simulink model "FCS_MPC_6ph_CIL_FCS_reduced"  (R2022a)
settings: Solver=ode23t  StartTime=0.0  StopTime=0.1  RelTol=1e-3  AbsTol=1e-3  EnableMultiTasking=on
values from neighbouring files (symbols this model uses):
  f_c = 100000    [Params_testbench.m]
  L_d = 0.0001473    [Params_testbench.m]
  L_q = 0.0001484    [Params_testbench.m]
  L_x = 0.00005566    (= 5.566e-05)    [Params_testbench.m]
  L_y = L_x    (= 5.566e-05)    [Params_testbench.m]
  p = 5    [Params_testbench.m]
  psi_pm = 0.0048    [Params_testbench.m]
  R_ph = 0.1278    [Params_testbench.m]
  u_dc = 36.0    (= 36)    [Params_testbench.m]
libraries: nesl_utility x39, fl_lib x32, hdlsllib x20, ee_lib x12, simulink x2, spsAlphaBetaZerotodq0Lib x1
(part 2 of 3)

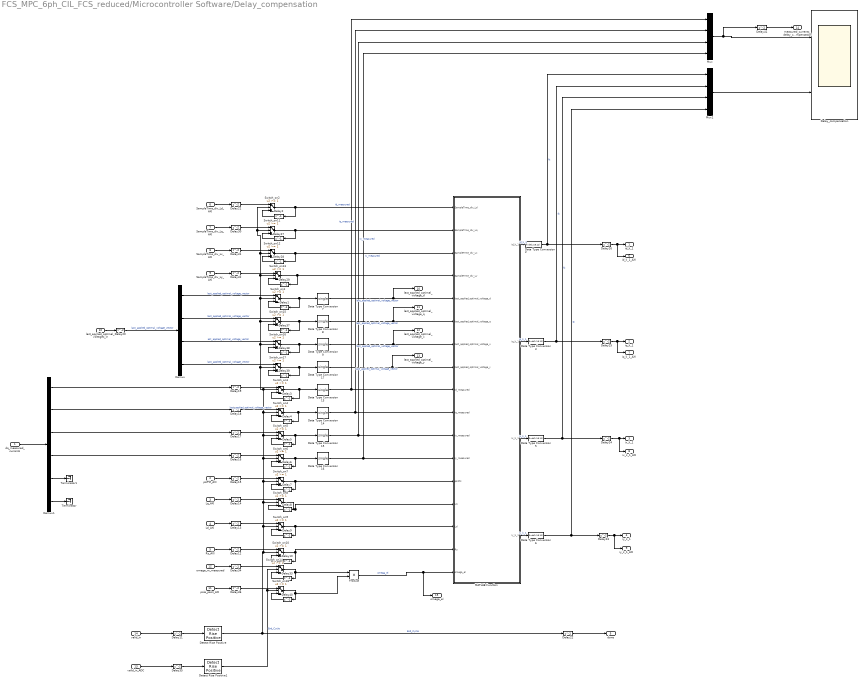
== system FCS_MPC_6ph_CIL_FCS_reduced/Microcontroller Software/Delay_compensation ==
  dq_measured_currents : Inport
  psiPM_AXI : Inport  Port=2
  Lq_AXI : Inport  Port=3
  Ld_AXI : Inport  Port=4
  Rs_AXI : Inport  Port=5
  SampleTime_div_Ld_AXI : Inport  Port=6
  SampleTime_div_Lq_AXI : Inport  Port=7
  SampleTime_div_Lx_AXI : Inport  Port=8
  SampleTime_div_Ly_AXI : Inport  Port=9
  last_applied_optimal_voltages_in : Inport  Port=10
  pole_pairs_AXI : Inport  Port=11
  omega_m_measured : Inport  Port=12
  valid_in_ADC : Inport  Port=13
  valid_in : Inport  Port=14
  Data Type Conversion{7..9,13..17} (8 alike) : DataTypeConversion  OutDataTypeStr=single  RndMeth=Nearest  SaturateOnIntegerOverflow=off
  Data Type Conversion{2..3,5..6} (4 alike) : DataTypeConversion  OutDataTypeStr=fixdt(1,18,11)  SaturateOnIntegerOverflow=off  RndMeth=Floor
  Delay{1..10,27..29,33,37..40} (18 alike) : Delay  DelayLength=1
  Delay{11..26,30..32,34..36,41} (23 alike) : Delay
  Delay_compensation : Scope  NumInputPorts=2
  Demux : Demux
  Demux1 : Demux  Outputs=6
  Detect Rise Positive : hdlsllib/Logic and Bit Operations/Detect Rise Positive  vinit=0  OutDataTypeStr=boolean
      settings: SourceProductBaseCode=SL
  Detect Rise Positive1 : hdlsllib/Logic and Bit Operations/Detect Rise Positive  vinit=0  OutDataTypeStr=boolean
      settings: SourceProductBaseCode=SL
  MATLAB Function : MATLAB Function  TreatAsAtomicUnit=on  SystemSampleTime=1/100000000
  Mux : Mux
  Mux1 : Mux
  Product : Product  Inputs=**
  Switch_on{1..18} (18 alike) : Switch  Threshold=1  RndMeth=Simplest  SaturateOnIntegerOverflow=off  InputSameDT=off  OutDataTypeStr=Inherit: Same as first input
  Terminator : Terminator
  Terminator1 : Terminator
  id_k_1 : Outport
  iq_k_1 : Outport  Port=2
  ix_k_1 : Outport  Port=3
  iy_k_1 : Outport  Port=4
  done : Outport  Port=5
  id_k_1_AXI : Outport  Port=6
  iq_k_1_AXI : Outport  Port=7
  ix_k_1_AXI : Outport  Port=8
  iy_k_1_AXI : Outport  Port=9
  last_applied_optimal_voltage_d : Outport  Port=10
  last_applied_optimal_voltage_q : Outport  Port=11
  last_applied_optimal_voltage_x : Outport  Port=12
  last_applied_optimal_voltage_y : Outport  Port=13
  measured_currents_delay_compensation : Outport  Port=14
  omega_el : Outport  Port=15
  wires:
  Delay33/1 -> Switch_on14/3
  pole_pairs_AXI/1 -> Delay36/1
  Delay9/1 -> Switch_on9/3
  Switch_on9/1 -> Delay9/1, MATLAB Function/15(Ld)
  Delay32/1 -> Switch_on13/1
  Lq_AXI/1 -> Delay14/1
  Delay31/1 -> Switch_on12/1
  Switch_on12/1 -> Delay28/1, MATLAB Function/3(SampleTime_div_Lx)
  Delay30/1 -> Switch_on11/1
  Delay29/1 -> Switch_on13/3
  SampleTime_div_Lx_AXI/1 -> Delay31/1
  Delay26/1 -> id_k_1_AXI/1, id_k_1/1
  Product/1 -> omega_el/1, MATLAB Function/17(omega_el)  "omega_el"
  Delay11/1 -> Detect Rise Positive/1
  Delay2/1 -> Switch_on2/3
  SampleTime_div_Lq_AXI/1 -> Delay30/1
  Switch_on5/1 -> Delay5/1, Data Type Conversion15/1
  Delay12/1 -> Switch_on10/1
  Rs_AXI/1 -> Delay12/1
  Delay1/1 -> Switch_on1/3
  Delay27/1 -> Switch_on11/3
  Delay21/1 -> Switch_on2/1
  Delay23/1 -> iy_k_1_AXI/1, iy_k_1/1
  Delay24/1 -> ix_k_1_AXI/1, ix_k_1/1
  Delay20/1 -> Demux/1  "last_applied_optimal_voltage_vector"
  Switch_on1/1 -> Delay1/1, Data Type Conversion7/1
  Delay8/1 -> Switch_on8/3
  Delay10/1 -> Switch_on10/3
  valid_in/1 -> Delay11/1
  Switch_on6/1 -> Delay6/1, Data Type Conversion16/1
  psiPM_AXI/1 -> Delay15/1
  Delay25/1 -> iq_k_1_AXI/1, iq_k_1/1
  Switch_on13/1 -> Delay29/1, MATLAB Function/4(SampleTime_div_Ly)
  Switch_on4/1 -> Delay4/1, Data Type Conversion14/1
  Delay15/1 -> Switch_on7/1
  SampleTime_div_Ly_AXI/1 -> Delay32/1
  Switch_on10/1 -> Delay10/1, MATLAB Function/16(Rs)
  Delay7/1 -> Switch_on7/3
  Delay28/1 -> Switch_on12/3
  Switch_on8/1 -> Delay8/1, MATLAB Function/14(Lq)
  Ld_AXI/1 -> Delay13/1
  Delay6/1 -> Switch_on6/3
  Delay4/1 -> Switch_on4/3
  Switch_on11/1 -> Delay27/1, MATLAB Function/2(SampleTime_div_Lq)
  Delay3/1 -> Switch_on3/3
  Delay14/1 -> Switch_on8/1
  Switch_on2/1 -> Delay2/1, MATLAB Function/1(SampleTime_div_Ld)
  Delay22/1 -> done/1
  Switch_on3/1 -> Delay3/1, Data Type Conversion13/1
  Delay13/1 -> Switch_on9/1
  Delay5/1 -> Switch_on5/3
  SampleTime_div_Ld_AXI/1 -> Delay21/1
  last_applied_optimal_voltages_in/1 -> Delay20/1
  omega_m_measured/1 -> Delay34/1
  Delay35/1 -> Detect Rise Positive1/1
  valid_in_ADC/1 -> Delay35/1
  Delay34/1 -> Switch_on14/1
  Delay36/1 -> Switch_on18/1
  Delay37/1 -> Switch_on15/3
  Delay38/1 -> Switch_on16/3
  Switch_on16/1 -> Data Type Conversion9/1, Delay38/1
  Delay39/1 -> Switch_on17/3
  Detect Rise Positive/1 -> Switch_on17/2, Switch_on16/2, Switch_on15/2, Switch_on13/2, Switch_on2/2, Switch_on11/2, Switch_on12/2, Switch_on1/2, Switch_on3/2, Switch_on4/2, Switch_on5/2, Switch_on6/2, Switch_on7/2, Switch_on8/2, Switch_on9/2, Switch_on10/2, Delay22/1  "End_Cycle"
  Switch_on17/1 -> Data Type Conversion17/1, Delay39/1
  Delay19/1 -> Switch_on3/1
  Delay18/1 -> Switch_on4/1  "last_applied_optimal_voltage_vector"
  Delay17/1 -> Switch_on5/1
  Delay16/1 -> Switch_on6/1
  Switch_on14/1 -> Product/1, Delay33/1
  MATLAB Function/1(id_k_1) -> Data Type Conversion2/1  "id_k_1"
  MATLAB Function/2(iq_k_1) -> Data Type Conversion3/1  "iq_k_1"
  MATLAB Function/3(ix_k_1) -> Data Type Conversion5/1  "ix_k_1"
  MATLAB Function/4(iy_k_1) -> Data Type Conversion6/1  "iy_k_1"
  Switch_on18/1 -> Product/2, Delay40/1
  Detect Rise Positive1/1 -> Switch_on18/2, Switch_on14/2  "End_Cycle"
  Delay40/1 -> Switch_on18/3
  Data Type Conversion13/1 -> Mux/1, MATLAB Function/9(id_measured)  "id_measured"
  Data Type Conversion14/1 -> Mux/2, MATLAB Function/10(iq_measured)  "iq_measured"
  Data Type Conversion15/1 -> Mux/3, MATLAB Function/11(ix_measured)  "ix_measured"
  Data Type Conversion16/1 -> Mux/4, MATLAB Function/12(iy_measured)  "iy_measured"
  Switch_on7/1 -> MATLAB Function/13(psiPM), Delay7/1
  Mux/1 -> Delay41/1, Delay_compensation/1
  Mux1/1 -> Delay_compensation/2
  Switch_on15/1 -> Data Type Conversion8/1, Delay37/1
  Demux/1 -> Switch_on1/1  "last_applied_optimal_voltage_vector"
  Demux/2 -> Switch_on15/1  "last_applied_optimal_voltage_vector"
  Demux/3 -> Switch_on16/1  "ast_applied_optimal_voltage_vector"
  Demux/4 -> Switch_on17/1  "last_applied_optimal_voltage_vector"
  Data Type Conversion2/1 -> Mux1/1, Delay26/1  "fc"
  Data Type Conversion3/1 -> Mux1/2, Delay25/1  "fc"
  Data Type Conversion5/1 -> Mux1/3, Delay24/1  "fc"
  Data Type Conversion6/1 -> Mux1/4, Delay23/1  "fc"
  Data Type Conversion7/1 -> last_applied_optimal_voltage_d/1, MATLAB Function/5(last_applied_optimal_voltage_d)  "last_applied_optimal_voltage_vector"
  Data Type Conversion8/1 -> last_applied_optimal_voltage_q/1, MATLAB Function/6(last_applied_optimal_voltage_q)  "last_applied_optimal_voltage_vector"
  Data Type Conversion9/1 -> last_applied_optimal_voltage_x/1, MATLAB Function/7(last_applied_optimal_voltage_x)  "last_applied_optimal_voltage_vector"
  Data Type Conversion17/1 -> last_applied_optimal_voltage_y/1, MATLAB Function/8(last_applied_optimal_voltage_y)  "last_applied_optimal_voltage_vector"
  Delay41/1 -> measured_currents_delay_compensation/1
  dq_measured_currents/1 -> Demux1/1
  Demux1/6 -> Terminator/1
  Demux1/5 -> Terminator1/1
  Demux1/1 -> Delay19/1
  Demux1/2 -> Delay18/1
  Demux1/3 -> Delay17/1
  Demux1/4 -> Delay16/1

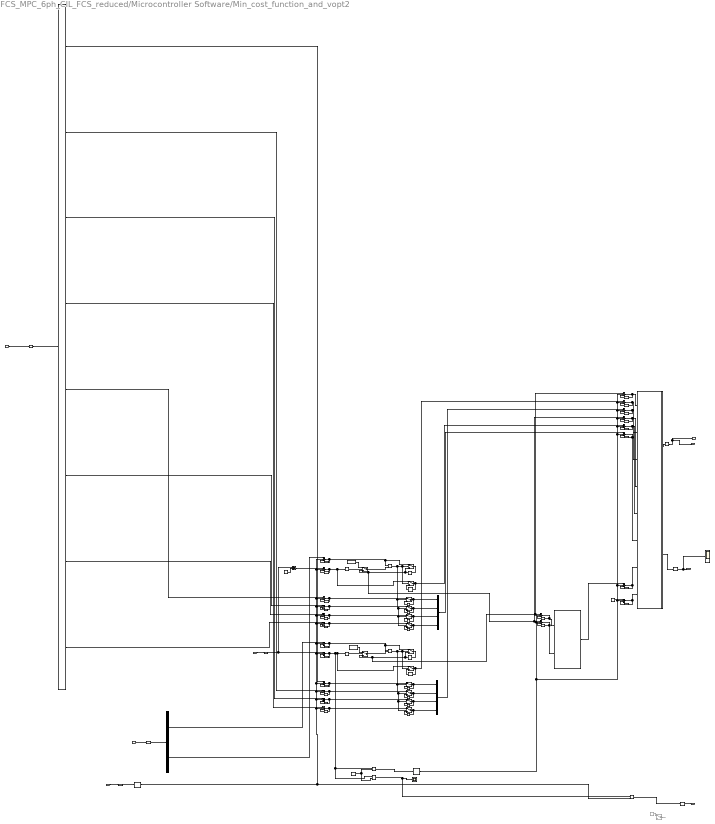
== system FCS_MPC_6ph_CIL_FCS_reduced/Microcontroller Software/Min_cost_function_and_vopt2 ==
  note: fixdt(1,24,11)
  Index_in : Inport
  valid_in : Inport  Port=2
  J_in : Inport  Port=3
  phase_voltages_per_switching_state_in : Inport  Port=4
  Add : Sum
  Compare To Constant : hdlsllib/Logic and Bit Operations/Compare To Constant  relop=<=  const=1  OutDataTypeStr=boolean
      settings: SourceProductBaseCode=SL
  Compare To Constant1 : hdlsllib/Logic and Bit Operations/Compare To Constant  relop=<=  const=9  OutDataTypeStr=boolean
      settings: SourceProductBaseCode=SL
  Constant : Constant  Value=1000  OutDataTypeStr=fixdt(1,20,9)  SampleTime=-1
  Constant1 : Constant  Value=8  OutDataTypeStr=int32  SampleTime=-1
  Constant11 : Constant  Value=[0;0;0;0]  OutDataTypeStr=fixdt(1,24,11)  SampleTime=-1
  Constant18 : Constant  Value=8  OutDataTypeStr=int32  SampleTime=-1
  Constant2 : Constant  Commented=on  Value=0  OutDataTypeStr=boolean  SampleTime=-1
  Constant3 : Constant  Value=1000  OutDataTypeStr=fixdt(1,20,9)  SampleTime=-1
  Delay{,1..5,9,15,17..23,25..26,34..43,56..57,68..71,371..372} (35 alike) : Delay  DelayLength=1
  Delay10 : Delay  DelayLength=3
  Delay11 : Delay  DelayLength=3
  Delay12 : Delay  DelayLength=3
  Delay6 : Delay
  Delay7 : Delay
  Delay8 : Delay
  Delay_compensation_test1 : Scope
  Demux : Demux  Outputs=2
  Demux1 : Demux  Outputs=8
  Detect Rise Positive : hdlsllib/Logic and Bit Operations/Detect Rise Positive  vinit=0  OutDataTypeStr=boolean
      settings: SourceProductBaseCode=SL
  Detect Rise Positive1 : hdlsllib/Logic and Bit Operations/Detect Rise Positive  vinit=0  OutDataTypeStr=boolean
      settings: SourceProductBaseCode=SL
  Logical Operator : Logic  AllPortsSameDT=off  OutDataTypeStr=boolean
  MATLAB Function : MATLAB Function  TreatAsAtomicUnit=on  SystemSampleTime=1/100000000
  MinMax : MinMax  Inputs=2  ZeroCross=off
  Mux : Mux
  Mux1 : Mux
  Relational Operator : RelationalOperator  Operator=<  OutDataTypeStr=boolean  RndMeth=Simplest  InputSameDT=off
  Relational Operator1 : RelationalOperator  Operator=<  OutDataTypeStr=boolean  RndMeth=Simplest  InputSameDT=off
  Relational Operator2 : RelationalOperator  Operator=<  OutDataTypeStr=boolean  RndMeth=Simplest  InputSameDT=off
  Relational Operator9 : RelationalOperator  OutDataTypeStr=boolean  RndMeth=Simplest  InputSameDT=off
  Scope : Scope
  Switch{,1,3..6,8..9,11..14} (12 alike) : Switch  Criteria=u2 > Threshold  SaturateOnIntegerOverflow=off  InputSameDT=off  OutDataTypeStr=Inherit: Same as first input
  Switch10 : Switch  Criteria=u2 > Threshold  OutDataTypeStr=int32  SaturateOnIntegerOverflow=off  InputSameDT=off
  Switch2 : Switch  Criteria=u2 > Threshold  OutDataTypeStr=int32  SaturateOnIntegerOverflow=off  InputSameDT=off
  Switch7 : Switch  Commented=on  Criteria=u2 > Threshold  SaturateOnIntegerOverflow=off  InputSameDT=off
  Switch_on{1..13,51,70..75,98..99} (22 alike) : Switch  Threshold=1  RndMeth=Simplest  SaturateOnIntegerOverflow=off  InputSameDT=off  OutDataTypeStr=Inherit: Same as first input
  done : Outport
  Index : Outport  Port=2
  voltages : Outport  Port=3
  Index_AXI : Outport  Port=4
  wires:
  Demux/1 -> Switch_on4/1  "End_Cycle"
  Demux1/1 -> Switch_on2/1  "End_Cycle"
  Demux1/2 -> Switch_on3/1  "End_Cycle"
  Switch5/1 -> Mux/3, Delay4/1
  Delay3/1 -> Switch4/3
  Relational Operator/1 -> Switch5/2, Switch6/2, Switch4/2, Switch3/2, Switch2/2, Switch1/2
  Compare To Constant/1 -> Switch/2
  Switch1/1 -> Delay/1
  Switch6/1 -> Delay5/1, Mux/4
  Delay4/1 -> Switch5/3
  Switch4/1 -> Mux/2, Delay3/1
  Switch/1 -> Relational Operator/2
  Delay1/1 -> Switch2/3
  Delay5/1 -> Switch6/3
  Switch3/1 -> Mux/1, Delay2/1
  Delay2/1 -> Switch3/3
  Constant/1 -> Switch/1
  Switch_on4/1 -> Relational Operator/1, Switch1/1, Delay17/1
  Switch_on1/1 -> Delay18/1, Compare To Constant/1, Switch2/1, Relational Operator9/1, Relational Operator1/1
  Switch_on2/1 -> Delay19/1, Switch3/1
  Switch_on3/1 -> Delay20/1, Switch4/1
  Switch_on5/1 -> Switch5/1, Delay21/1
  Switch_on6/1 -> Switch6/1, Delay22/1
  valid_in/1 -> Delay6/1  "End_Cycle"
  Delay17/1 -> Switch_on4/3
  Delay18/1 -> Switch_on1/3
  Delay19/1 -> Switch_on2/3
  Delay20/1 -> Switch_on3/3
  Delay21/1 -> Switch_on5/3
  Delay22/1 -> Switch_on6/3
  Constant1/1 -> Relational Operator9/2, Relational Operator1/2
  Constant2/1 -> Switch7/1
  Demux1/3 -> Switch_on5/1  "End_Cycle"
  Demux1/4 -> Switch_on6/1  "End_Cycle"
  Demux/2 -> Switch_on10/1  "End_Cycle"
  Delay34/1 -> Switch_on10/3
  Switch8/1 -> Relational Operator2/2
  Switch_on8/1 -> Delay36/1, Switch11/1
  Demux1/6 -> Switch_on9/1  "End_Cycle"
  Delay26/1 -> Switch10/3
  Add/1 -> Switch_on7/1
  Delay36/1 -> Switch_on8/3
  Delay39/1 -> Switch_on11/3
  Switch_on7/1 -> Delay35/1, Switch10/1, Compare To Constant1/1
  Compare To Constant1/1 -> Switch8/2
  Switch_on9/1 -> Delay38/1, Switch12/1
  Delay40/1 -> Switch_on12/3
  Delay35/1 -> Switch_on7/3
  Switch_on11/1 -> Switch13/1, Delay39/1
  Delay43/1 -> Switch14/3
  Switch_on12/1 -> Switch14/1, Delay40/1
  Delay37/1 -> Switch11/3
  Relational Operator2/1 -> Switch13/2, Switch14/2, Switch12/2, Switch11/2, Switch10/2, Switch9/2
  Switch9/1 -> Delay25/1
  Delay42/1 -> Switch13/3
  Demux1/5 -> Switch_on8/1  "End_Cycle"
  Demux1/7 -> Switch_on11/1  "End_Cycle"
  Switch_on10/1 -> Relational Operator2/1, Switch9/1, Delay34/1
  Demux1/8 -> Switch_on12/1  "End_Cycle"
  Delay38/1 -> Switch_on9/3
  Constant3/1 -> Switch8/1
  Delay41/1 -> Switch12/3
  Detect Rise Positive/1 -> Logical Operator/2, Switch_on10/2, Switch_on7/2, Switch_on8/2, Switch_on9/2, Switch_on11/2, Switch_on12/2, Switch_on4/2, Switch_on1/2, Switch_on2/2, Switch_on3/2, Switch_on5/2, Switch_on6/2  "End_Cycle"
  Constant18/1 -> Add/2
  Delay371/1 -> Switch_on98/3
  Switch_on98/1 -> Delay371/1, MinMax/1
  Switch_on99/1 -> Delay372/1, MinMax/2
  Delay372/1 -> Switch_on99/3
  Relational Operator1/1 -> Logical Operator/1, Scope/1  "End_Cycle"
  Switch13/1 -> Mux1/3, Delay42/1
  Switch12/1 -> Mux1/2, Delay41/1
  Switch14/1 -> Mux1/4, Delay43/1
  Switch11/1 -> Mux1/1, Delay37/1
  J_in/1 -> Delay7/1  "End_Cycle"
  phase_voltages_per_switching_state_in/1 -> Delay8/1  "End_Cycle"
  Logical Operator/1 -> Delay12/1
  Delay6/1 -> Detect Rise Positive/1
  Delay7/1 -> Demux/1
  Delay8/1 -> Demux1/1
  Index_in/1 -> Delay9/1
  Switch7/1 -> ?
  MATLAB Function/2(voltages) -> Delay11/1
  MATLAB Function/1(Index) -> Delay10/1
  Constant11/1 -> Switch_on13/1
  Switch_on13/1 -> MATLAB Function/8(voltages_default), Delay15/1
  Delay15/1 -> Switch_on13/3
  Switch_on51/1 -> MATLAB Function/7(min), Delay23/1
  Delay23/1 -> Switch_on51/3
  Switch_on70/1 -> MATLAB Function/6(voltages_2), Delay56/1
  Delay56/1 -> Switch_on70/3
  Switch10/1 -> Switch_on71/1, Delay26/1
  Switch_on71/1 -> MATLAB Function/5(Index_2), Delay57/1
  Delay57/1 -> Switch_on71/3
  Switch_on72/1 -> MATLAB Function/4(J_2), Delay68/1
  Delay68/1 -> Switch_on72/3
  Switch_on73/1 -> MATLAB Function/3(voltages_1), Delay69/1
  Delay69/1 -> Switch_on73/3
  Switch2/1 -> Switch_on74/1, Delay1/1
  Switch_on74/1 -> MATLAB Function/2(Index_1), Delay70/1
  Delay70/1 -> Switch_on74/3
  Switch_on75/1 -> MATLAB Function/1(J_1), Delay71/1
  Delay71/1 -> Switch_on75/3
  Delay/1 -> Switch_on75/1, Switch_on98/1, Switch/3, Switch1/3  "last_applied_optimal_voltage_vector"
  Mux/1 -> Switch_on73/1  "last_applied_optimal_voltage_vector"
  Delay25/1 -> Switch_on72/1, Switch_on99/1, Switch8/3, Switch9/3  "last_applied_optimal_voltage_vector"
  Mux1/1 -> Switch_on70/1  "last_applied_optimal_voltage_vector"
  MinMax/1 -> Switch_on51/1  "last_applied_optimal_voltage_vector"
  Delay10/1 -> Index_AXI/1, Index/1
  Delay11/1 -> Delay_compensation_test1/1, voltages/1
  Delay12/1 -> done/1
  Detect Rise Positive1/1 -> Switch_on75/2, Switch_on74/2, Switch_on73/2, Switch_on72/2, Switch_on71/2, Switch_on70/2, Switch_on51/2, Switch_on13/2, Switch_on98/2, Switch_on99/2  "End_Cycle"
  Relational Operator9/1 -> Detect Rise Positive1/1  "End_Cycle"
  Delay9/1 -> Switch_on1/1, Add/1

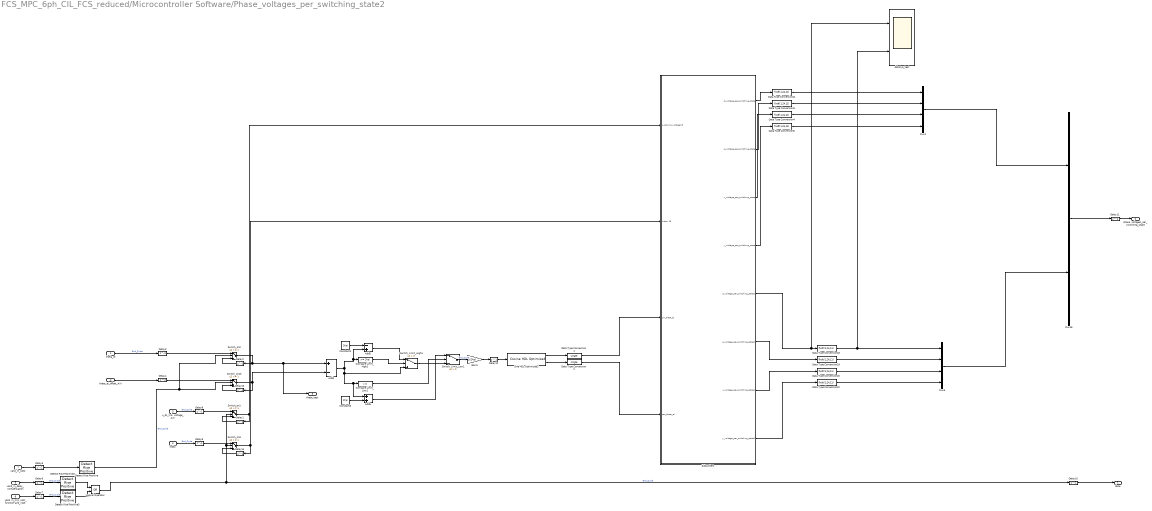
== system FCS_MPC_6ph_CIL_FCS_reduced/Microcontroller Software/Phase_voltages_per_switching_state2 ==
  theta_el : Inport
  theta_el_offset_AXI : Inport  Port=2
  u_dc_link_voltage_AXI : Inport  Port=3
  Index : Inport  Port=4
  valid_in_delay_compensation : Inport  Port=5
  valid_in_min_cost_function-and_vopt : Inport  Port=6
  valid_in_ADC : Inport  Port=7
  Add4 : Sum  Inputs=+-  OutDataTypeStr=Inherit: Same as first input
  Add5 : Sum  Inputs=-+  OutDataTypeStr=Inherit: Same as first input
  Add6 : Sum  OutDataTypeStr=Inherit: Same as first input
  Compare Limit_High1 : simulink/Logic and Bit Operations/Compare To Constant  relop=>=  const=2*pi  OutDataTypeStr=boolean
  Compare Limit_Low1 : simulink/Logic and Bit Operations/Compare To Constant  relop=<  const=0  OutDataTypeStr=boolean
  Constant2 : Constant  Value=2*pi  OutDataTypeStr=fixdt(1,18,14)  SampleTime=1/100000000
  Constant3 : Constant  Value=2*pi  OutDataTypeStr=fixdt(1,18,14)  SampleTime=1/100000000
  Data Type Conversion1 : DataTypeConversion  OutDataTypeStr=single  SaturateOnIntegerOverflow=off  RndMeth=Floor
  Data Type Conversion{3..5,18..22} (8 alike) : DataTypeConversion  OutDataTypeStr=fixdt(1,24,11)  SaturateOnIntegerOverflow=off  RndMeth=Floor
  Data Type Conversion2 : DataTypeConversion  OutDataTypeStr=single  SaturateOnIntegerOverflow=off  RndMeth=Floor
  Delay{1..2,6..14} (11 alike) : Delay  DelayLength=1
  Delay3 : Delay
  Delay4 : Delay
  Delay5 : Delay
  Detect Rise Positive : hdlsllib/Logic and Bit Operations/Detect Rise Positive  vinit=0  OutDataTypeStr=boolean
      settings: SourceProductBaseCode=SL
  Detect Rise Positive2 : hdlsllib/Logic and Bit Operations/Detect Rise Positive  vinit=0  OutDataTypeStr=boolean
      settings: SourceProductBaseCode=SL
  Detect Rise Positive3 : hdlsllib/Logic and Bit Operations/Detect Rise Positive  vinit=0  OutDataTypeStr=boolean
      settings: SourceProductBaseCode=SL
  Gain1 : Gain  Gain=1/(2*pi)  OutDataTypeStr=Inherit: Same as input  ParamDataTypeStr=Inherit: Same as input
  Logical Operator : Logic  Operator=OR  AllPortsSameDT=off  OutDataTypeStr=boolean
  Mux1 : Mux
  Mux16 : Mux  Inputs=2
  Mux5 : Mux
  Sine HDL Optimized2 : hdlsllib/Lookup Tables/Cosine HDL Optimized  OutputFormula=sin(2*pi*u) and cos(2*pi*u)  NumDataPoints=512  TableDataTypeStr=fixdt(1,15,14)  SimulateLUTROMDelay=off
      settings: SourceProductBaseCode=SL
  Subsystem : Subsystem
  Switch_Limit_High1 : Switch  Criteria=u2 > Threshold  SaturateOnIntegerOverflow=off  InputSameDT=off  OutDataTypeStr=Inherit: Same as first input
  Switch_Limit_Low1 : Switch  Criteria=u2 > Threshold  SaturateOnIntegerOverflow=off  InputSameDT=off  OutDataTypeStr=Inherit: Same as first input
  Switch_on1 : Switch  Threshold=1  OutDataTypeStr=single  RndMeth=Simplest  SaturateOnIntegerOverflow=off  InputSameDT=off
  Switch_on13 : Switch  Threshold=1  RndMeth=Simplest  SaturateOnIntegerOverflow=off  InputSameDT=off  OutDataTypeStr=Inherit: Same as first input
  Switch_on2 : Switch  Threshold=1  RndMeth=Simplest  SaturateOnIntegerOverflow=off  InputSameDT=off  OutDataTypeStr=Inherit: Same as first input
  Switch_on3 : Switch  Threshold=1  OutDataTypeStr=int32  RndMeth=Simplest  SaturateOnIntegerOverflow=off  InputSameDT=off
  datatyp_test : Scope  NumInputPorts=2
  done : Outport
  phase_voltages_per_switching_state : Outport  Port=2
  theta_test : Outport  Port=3
  wires:
  Delay14/1 -> Switch_on3/3
  Delay13/1 -> Switch_on13/3
  Switch_on13/1 -> Delay13/1, Add4/2
  u_dc_link_voltage_AXI/1 -> Delay8/1  "End_Cycle"
  Switch_on1/1 -> Subsystem/1(u_dc_link_voltage15), Delay1/1
  Logical Operator/1 -> Delay10/1, Switch_on3/2, Switch_on1/2  "End_Cycle"
  Delay1/1 -> Switch_on1/3
  Index/1 -> Delay9/1  "End_Cycle"
  Switch_on3/1 -> Delay14/1, Subsystem/2(Index 15)
  Mux1/1 -> Mux16/1
  Mux5/1 -> Mux16/2
  Mux16/1 -> Delay11/1
  valid_in_ADC/1 -> Delay5/1
  valid_in_delay_compensation/1 -> Delay6/1
  valid_in_min_cost_function-and_vopt/1 -> Delay7/1
  theta_el/1 -> Delay3/1  "End_Cycle"
  Add4/1 -> Switch_Limit_High1/3, Add6/1, Compare Limit_Low1/1, Add5/2, Compare Limit_High1/1
  Compare Limit_Low1/1 -> Switch_Limit_Low1/2
  Add5/1 -> Switch_Limit_High1/1
  theta_el_offset_AXI/1 -> Delay4/1
  Constant3/1 -> Add6/2
  Constant2/1 -> Add5/1
  Compare Limit_High1/1 -> Switch_Limit_High1/2
  Add6/1 -> Switch_Limit_Low1/1
  Switch_Limit_High1/1 -> Switch_Limit_Low1/3
  Delay2/1 -> Switch_on2/3
  Switch_on2/1 -> theta_test/1, Add4/1, Delay2/1
  Detect Rise Positive/1 -> Switch_on2/2, Switch_on13/2  "End_Cycle"
  Delay3/1 -> Switch_on2/1
  Delay4/1 -> Switch_on13/1
  Delay5/1 -> Detect Rise Positive/1
  Delay6/1 -> Detect Rise Positive2/1
  Delay7/1 -> Detect Rise Positive3/1
  Delay8/1 -> Switch_on1/1
  Delay9/1 -> Switch_on3/1
  Delay10/1 -> done/1
  Delay11/1 -> phase_voltages_per_switching_state/1
  Sine HDL Optimized2/2 -> Data Type Conversion2/1
  Subsystem/1(d_voltage_per_switching_state) -> Data Type Conversion21/1
  Subsystem/2(q_voltage_per_switching_state) -> Data Type Conversion3/1
  Subsystem/3(x_voltage_per_switching_state) -> Data Type Conversion4/1
  Subsystem/4(y_voltage_per_switching_state) -> Data Type Conversion5/1
  Subsystem/5(d_voltage_per_switching_state2) -> datatyp_test/1, Data Type Conversion18/1
  Subsystem/6(q_voltage_per_switching_state2) -> Data Type Conversion19/1
  Subsystem/7(x_voltage_per_switching_state2) -> Data Type Conversion20/1
  Subsystem/8(y_voltage_per_switching_state2) -> Data Type Conversion22/1
  Gain1/1 -> Delay12/1
  Switch_Limit_Low1/1 -> Gain1/1  "End_Cycle"
  Data Type Conversion21/1 -> Mux1/1
  Data Type Conversion3/1 -> Mux1/2
  Data Type Conversion4/1 -> Mux1/3
  Data Type Conversion5/1 -> Mux1/4
  Data Type Conversion18/1 -> datatyp_test/2, Mux5/1
  Data Type Conversion19/1 -> Mux5/2
  Data Type Conversion20/1 -> Mux5/3
  Data Type Conversion22/1 -> Mux5/4
  Detect Rise Positive2/1 -> Logical Operator/1  "End_Cycle"
  Detect Rise Positive3/1 -> Logical Operator/2  "End_Cycle"
  Data Type Conversion2/1 -> Subsystem/4(cos_theta_el)
  Sine HDL Optimized2/1 -> Data Type Conversion1/1
  Data Type Conversion1/1 -> Subsystem/3(sin_theta_el)
  Delay12/1 -> Sine HDL Optimized2/1

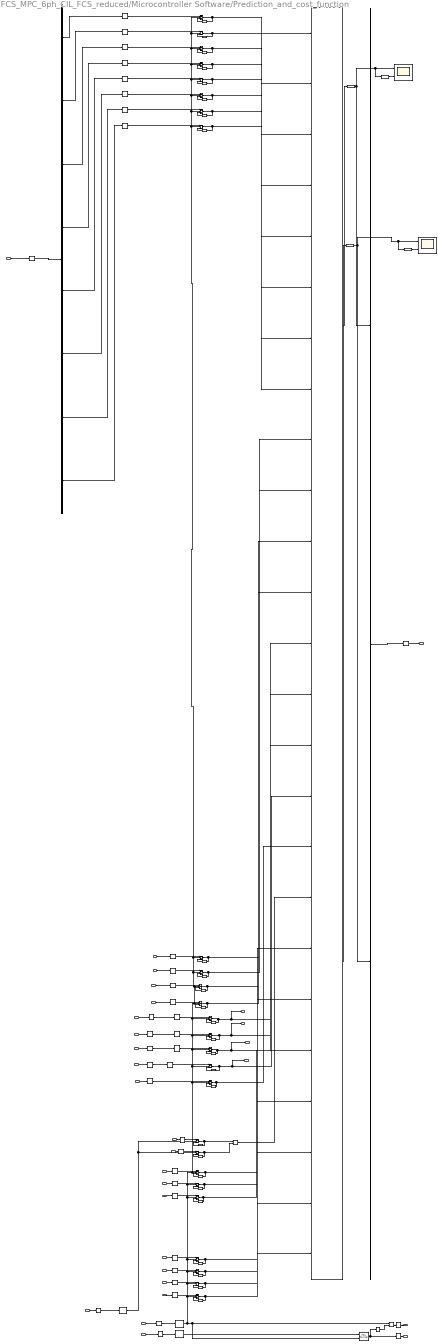
== system FCS_MPC_6ph_CIL_FCS_reduced/Microcontroller Software/Prediction_and_cost_function ==
  Lq_AXI : Inport
  Ld_AXI : Inport  Port=2
  SampleTime_div_Ld_AXI : Inport  Port=3
  SampleTime_div_Lq_AXI : Inport  Port=4
  SampleTime_div_Lx_AXI : Inport  Port=5
  SampleTime_div_Ly_AXI : Inport  Port=6
  id_k_1 : Inport  Port=7
  iq_k_1 : Inport  Port=8
  ix_k_1 : Inport  Port=9
  iy_k_1 : Inport  Port=10
  Rs_AXI : Inport  Port=11
  omega_m_measured : Inport  Port=12
  pole_pairs_AXI : Inport  Port=13
  psiPM_AXI : Inport  Port=14
  id_ref_AXI : Inport  Port=15
  iq_ref_AXI : Inport  Port=16
  ix_ref_AXI : Inport  Port=17
  iy_ref_AXI : Inport  Port=18
  valid_in : Inport  Port=19
  Reset : Inport  Port=20
  valid_in_ADC : Inport  Port=21
  dqxy_phase_voltage_per_switching_state : Inport  Port=22
  Compare To Constant : hdlsllib/Logic and Bit Operations/Compare To Constant  relop=<=  const=8  OutDataTypeStr=boolean
      settings: SourceProductBaseCode=SL
  Data Type Conversion{1..3,5..13} (12 alike) : DataTypeConversion  OutDataTypeStr=single  RndMeth=Nearest  SaturateOnIntegerOverflow=off
  Data Type Conversion{18,39,46,54} (4 alike) : DataTypeConversion  OutDataTypeStr=fixdt(1,20,9)  SaturateOnIntegerOverflow=off  RndMeth=Floor
  Delay{,5..7,21..32,34..42} (25 alike) : Delay
  Delay{1..4,8..20,33,128..135} (26 alike) : Delay  DelayLength=1
  Demux : Demux  Outputs=8
  Detect Rise Positive : hdlsllib/Logic and Bit Operations/Detect Rise Positive  vinit=0  OutDataTypeStr=boolean
      settings: SourceProductBaseCode=SL
  Detect Rise Positive1 : hdlsllib/Logic and Bit Operations/Detect Rise Positive  vinit=0  OutDataTypeStr=boolean
      settings: SourceProductBaseCode=SL
  Detect Rise Positive2 : hdlsllib/Logic and Bit Operations/Detect Rise Positive  vinit=0  OutDataTypeStr=boolean
      settings: SourceProductBaseCode=SL
  HDL Counter : hdlsllib/Sources/HDL Counter  CountType=Free running  CountInit=0  CountStep=1  CountMax=25  CountFromType=Initial value  CountFrom=0  CountResetPort=on  CountLoadPort=off  CountEnbPort=on  CountDirPort=off  CountHitOutputPort=off  CountDataType=Signed  CountWordLen=32  CountFracLen=0  CountSampTime=1
  J_fixed_point : Scope  NumInputPorts=2
  J_fixed_point1 : Scope  NumInputPorts=2
  Logical Operator : Logic  AllPortsSameDT=off  OutDataTypeStr=boolean
  Mux : Mux  Inputs=2
  Product : Product  Inputs=**
  Subsystem : Subsystem
  Switch_on{1..4,8..10,12..21,83..90} (25 alike) : Switch  Threshold=1  OutDataTypeStr=single  RndMeth=Simplest  SaturateOnIntegerOverflow=off  InputSameDT=off
  Switch_on11 : Switch  Threshold=1  RndMeth=Simplest  SaturateOnIntegerOverflow=off  InputSameDT=off  OutDataTypeStr=Inherit: Same as first input
  done : Outport
  Index : Outport  Port=2
  J : Outport  Port=3
  id_k_1_Prediction : Outport  Port=4
  iq_k_1_Prediction : Outport  Port=5
  ix_k_1_Prediction : Outport  Port=6
  iy_k_1_Prediction : Outport  Port=7
  wires:
  Switch_on12/1 -> Subsystem/17(Rs15), Delay12/1
  Rs_AXI/1 -> Delay26/1
  SampleTime_div_Ld_AXI/1 -> Delay5/1
  Delay3/1 -> Switch_on3/3
  Delay10/1 -> Switch_on10/3
  iq_ref_AXI/1 -> Delay34/1
  Delay17/1 -> Switch_on18/3
  Switch_on10/1 -> Delay10/1, Subsystem/19(Lq15)
  Delay11/1 -> Switch_on11/3
  SampleTime_div_Lq_AXI/1 -> Delay6/1
  Ld_AXI/1 -> Delay30/1
  psiPM_AXI/1 -> Delay31/1
  Delay1/1 -> Switch_on1/3
  id_ref_AXI/1 -> Delay32/1
  Product/1 -> Subsystem/18(omega_el15)  "omega_el"
  Delay9/1 -> Switch_on9/3
  Delay20/1 -> Switch_on21/3
  pole_pairs_AXI/1 -> Delay28/1
  Switch_on18/1 -> Delay17/1, Subsystem/12(SampleTime_div_Ly15)
  Delay19/1 -> Switch_on20/3
  Delay13/1 -> Switch_on13/3
  Switch_on15/1 -> Delay14/1, ix_k_1_Prediction/1, Subsystem/15(ix_k_16)
  Delay18/1 -> Switch_on19/3
  Switch_on19/1 -> Delay18/1, Subsystem/11(SampleTime_div_Lx15)
  Switch_on20/1 -> Delay19/1, Subsystem/10(SampleTime_div_Lq15)
  Switch_on13/1 -> Delay13/1, iy_k_1_Prediction/1, Subsystem/16(iy_k_16)
  iy_ref_AXI/1 -> Delay36/1
  Delay2/1 -> Switch_on2/3
  Delay16/1 -> Switch_on17/3
  Switch_on17/1 -> Delay16/1, id_k_1_Prediction/1, Subsystem/13(id_k_16)
  Delay15/1 -> Switch_on16/3
  Switch_on16/1 -> Delay15/1, iq_k_1_Prediction/1, Subsystem/14(iq_k_16)
  Delay33/1 -> Switch_on14/3
  SampleTime_div_Lx_AXI/1 -> Delay7/1
  Switch_on14/1 -> Delay33/1, Subsystem/25(iy_ref15)
  Delay12/1 -> Switch_on12/3
  valid_in/1 -> Delay38/1
  Switch_on3/1 -> Delay3/1, Subsystem/22(id_ref15)
  Switch_on21/1 -> Delay20/1, Subsystem/9(SampleTime_div_Ld15)
  Switch_on2/1 -> Delay2/1, Subsystem/23(iq_ref15)
  Lq_AXI/1 -> Delay29/1
  Switch_on1/1 -> Delay1/1, Subsystem/24(ix_ref15)
  Switch_on9/1 -> Delay9/1, Subsystem/20(Ld15)
  SampleTime_div_Ly_AXI/1 -> Delay21/1
  Delay14/1 -> Switch_on15/3
  ix_ref_AXI/1 -> Delay35/1
  Switch_on8/1 -> Delay8/1, Subsystem/21(psiPM15)
  Delay8/1 -> Switch_on8/3
  id_k_1/1 -> Delay22/1
  iq_k_1/1 -> Delay23/1
  ix_k_1/1 -> Delay24/1
  iy_k_1/1 -> Delay25/1
  omega_m_measured/1 -> Delay27/1
  Reset/1 -> Delay39/1
  Detect Rise Positive1/1 -> HDL Counter/1  "End_Cycle"
  Compare To Constant/1 -> Logical Operator/2
  HDL Counter/1 -> Delay41/1, Compare To Constant/1
  valid_in_ADC/1 -> Delay37/1
  Mux/1 -> Delay42/1
  Switch_on85/1 -> Subsystem/6(q_phase_voltage_per_switching_state1), Delay130/1
  Delay130/1 -> Switch_on85/3
  Delay131/1 -> Switch_on86/3
  Switch_on86/1 -> Subsystem/5(d_phase_voltage_per_switching_state1), Delay131/1
  Delay128/1 -> Switch_on83/3
  Switch_on83/1 -> Subsystem/8(y_phase_voltage_per_switching_state1), Delay128/1
  Delay129/1 -> Switch_on84/3
  Switch_on84/1 -> Subsystem/7(x_phase_voltage_per_switching_state1), Delay129/1
  Switch_on89/1 -> Subsystem/2(q_phase_voltage_per_switching_state), Delay134/1
  Delay134/1 -> Switch_on89/3
  Delay135/1 -> Switch_on90/3
  Switch_on90/1 -> Subsystem/1(d_phase_voltage_per_switching_state), Delay135/1
  Delay132/1 -> Switch_on87/3
  Switch_on87/1 -> Subsystem/4(y_phase_voltage_per_switching_state), Delay132/1
  Delay133/1 -> Switch_on88/3
  Switch_on88/1 -> Subsystem/3(x_phase_voltage_per_switching_state), Delay133/1
  Detect Rise Positive/1 -> Logical Operator/1, HDL Counter/2, Switch_on14/2, Switch_on1/2, Switch_on8/2, Switch_on9/2, Switch_on12/2, Switch_on20/2, Switch_on90/2, Switch_on89/2, Switch_on88/2, Switch_on87/2, Switch_on86/2, Switch_on85/2, Switch_on84/2, Switch_on83/2, Switch_on21/2, Switch_on19/2, Switch_on18/2, Switch_on17/2, Switch_on16/2, Switch_on15/2, Switch_on13/2, Switch_on10/2, Switch_on3/2, Switch_on2/2  "End_Cycle"
  Demux/8 -> Data Type Conversion13/1
  Demux/7 -> Data Type Conversion12/1
  Demux/6 -> Data Type Conversion11/1
  Demux/5 -> Data Type Conversion6/1
  Demux/4 -> Data Type Conversion5/1
  Demux/3 -> Data Type Conversion3/1
  Demux/2 -> Data Type Conversion2/1
  Demux/1 -> Data Type Conversion1/1
  Logical Operator/1 -> Delay40/1
  dqxy_phase_voltage_per_switching_state/1 -> Delay/1
  Data Type Conversion10/1 -> Switch_on13/1
  Data Type Conversion9/1 -> Switch_on15/1
  Data Type Conversion8/1 -> Switch_on16/1
  Data Type Conversion7/1 -> Switch_on17/1
  Switch_on11/1 -> Product/1, Delay11/1
  Data Type Conversion13/1 -> Switch_on83/1
  Data Type Conversion12/1 -> Switch_on84/1
  Data Type Conversion11/1 -> Switch_on85/1
  Data Type Conversion6/1 -> Switch_on86/1
  Data Type Conversion5/1 -> Switch_on87/1
  Data Type Conversion3/1 -> Switch_on88/1
  Data Type Conversion2/1 -> Switch_on89/1
  Data Type Conversion1/1 -> Switch_on90/1
  Detect Rise Positive2/1 -> Switch_on4/2, Switch_on11/2  "End_Cycle"
  Switch_on4/1 -> Product/2, Delay4/1
  Delay4/1 -> Switch_on4/3
  Data Type Conversion18/1 -> J_fixed_point/2  "fc"
  Data Type Conversion39/1 -> J_fixed_point1/2  "fc"
  Subsystem/2(J1) -> Data Type Conversion46/1  "fc"
  Subsystem/1(J) -> Data Type Conversion54/1  "fc"
  Data Type Conversion54/1 -> Data Type Conversion18/1, J_fixed_point/1, Mux/1  "fc"
  Data Type Conversion46/1 -> Data Type Conversion39/1, J_fixed_point1/1, Mux/2  "fc"
  Delay/1 -> Demux/1
  Delay5/1 -> Switch_on21/1
  Delay6/1 -> Switch_on20/1
  Delay7/1 -> Switch_on19/1
  Delay21/1 -> Switch_on18/1
  Delay22/1 -> Data Type Conversion7/1
  Delay23/1 -> Data Type Conversion8/1
  Delay24/1 -> Data Type Conversion9/1
  Delay25/1 -> Data Type Conversion10/1
  Delay26/1 -> Switch_on12/1
  Delay27/1 -> Switch_on11/1
  Delay28/1 -> Switch_on4/1
  Delay29/1 -> Switch_on10/1
  Delay30/1 -> Switch_on9/1
  Delay31/1 -> Switch_on8/1
  Delay32/1 -> Switch_on3/1
  Delay34/1 -> Switch_on2/1
  Delay35/1 -> Switch_on1/1
  Delay36/1 -> Switch_on14/1
  Delay37/1 -> Detect Rise Positive2/1
  Delay38/1 -> Detect Rise Positive/1
  Delay39/1 -> Detect Rise Positive1/1
  Delay40/1 -> done/1
  Delay41/1 -> Index/1
  Delay42/1 -> J/1

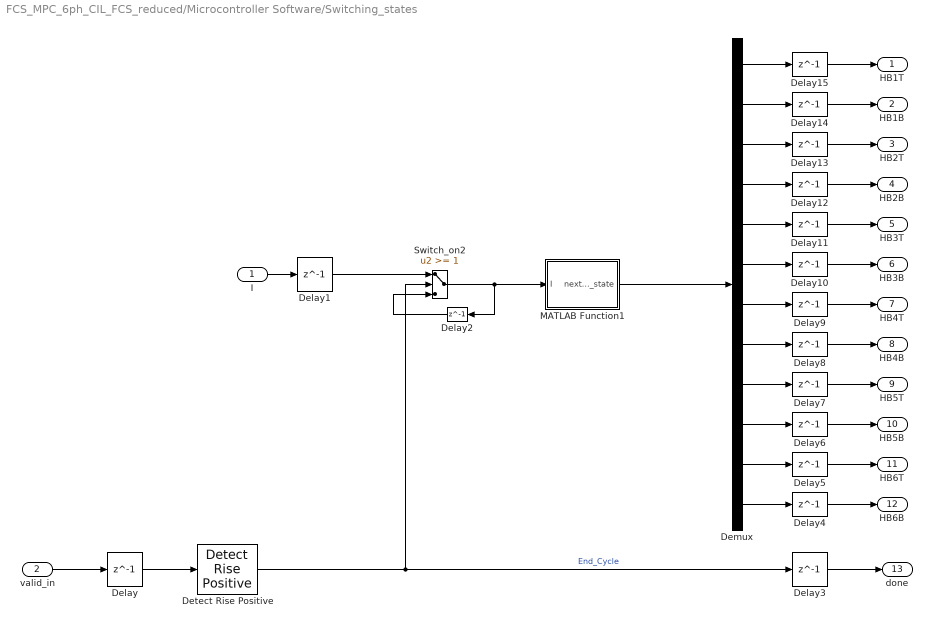
== system FCS_MPC_6ph_CIL_FCS_reduced/Microcontroller Software/Switching_states ==
  I : Inport
  valid_in : Inport  Port=2
  Delay{,1..15} (16 alike) : Delay  DelayLength=1
  Demux : Demux  Outputs=12
  Detect Rise Positive : hdlsllib/Logic and Bit Operations/Detect Rise Positive  vinit=0  OutDataTypeStr=boolean
      settings: SourceProductBaseCode=SL
  MATLAB Function1 : MATLAB Function  TreatAsAtomicUnit=on
  Switch_on2 : Switch  Threshold=1  OutDataTypeStr=Inherit: Inherit via back propagation  RndMeth=Simplest  SaturateOnIntegerOverflow=off  InputSameDT=off
  HB1T : Outport
  HB1B : Outport  Port=2
  HB2T : Outport  Port=3
  HB2B : Outport  Port=4
  HB3T : Outport  Port=5
  HB3B : Outport  Port=6
  HB4T : Outport  Port=7
  HB4B : Outport  Port=8
  HB5T : Outport  Port=9
  HB5B : Outport  Port=10
  HB6T : Outport  Port=11
  HB6B : Outport  Port=12
  done : Outport  Port=13
  wires:
  Demux/4 -> Delay12/1
  I/1 -> Delay1/1
  Demux/6 -> Delay10/1
  Demux/12 -> Delay4/1
  Demux/8 -> Delay8/1
  valid_in/1 -> Delay/1
  Demux/7 -> Delay9/1
  Demux/2 -> Delay14/1
  Detect Rise Positive/1 -> Delay3/1, Switch_on2/2  "End_Cycle"
  Demux/5 -> Delay11/1
  Delay2/1 -> Switch_on2/3
  Demux/1 -> Delay15/1
  Demux/9 -> Delay7/1
  Demux/10 -> Delay6/1
  MATLAB Function1/1(next_switching_state) -> Demux/1
  Demux/3 -> Delay13/1
  Delay/1 -> Detect Rise Positive/1
  Delay1/1 -> Switch_on2/1
  Delay3/1 -> done/1
  Delay4/1 -> HB6B/1
  Demux/11 -> Delay5/1
  Delay5/1 -> HB6T/1
  Delay6/1 -> HB5B/1
  Delay7/1 -> HB5T/1
  Delay8/1 -> HB4B/1
  Delay9/1 -> HB4T/1
  Delay10/1 -> HB3B/1
  Delay11/1 -> HB3T/1
  Delay12/1 -> HB2B/1
  Delay13/1 -> HB2T/1
  Delay14/1 -> HB1B/1
  Delay15/1 -> HB1T/1
  Switch_on2/1 -> MATLAB Function1/1(I), Delay2/1

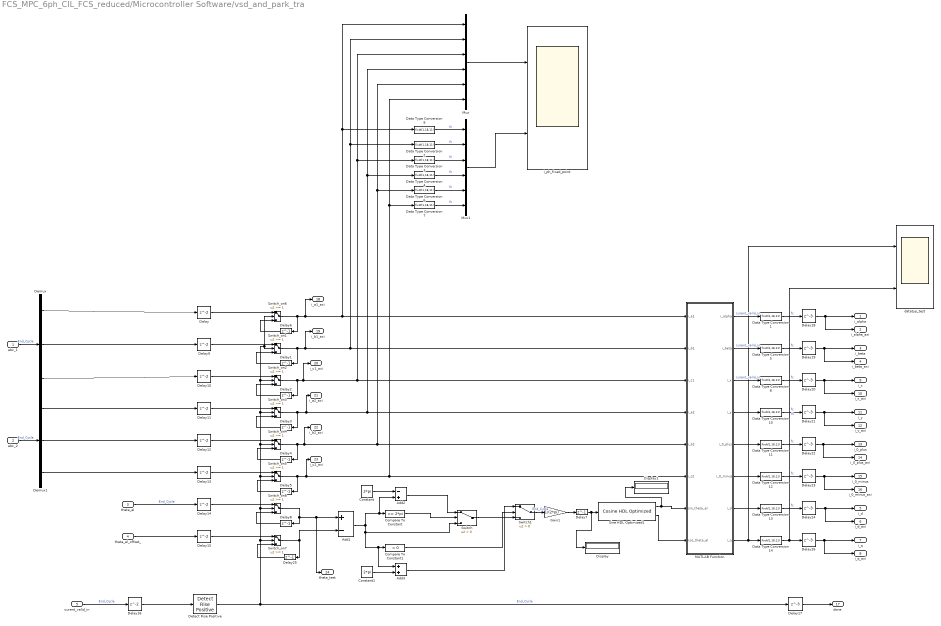
== system FCS_MPC_6ph_CIL_FCS_reduced/Microcontroller Software/vsd_and_park_tra ==
  abc_1 : Inport
  abc_2 : Inport  Port=2
  theta_el : Inport  Port=3
  theta_el_offset_ : Inport  Port=4
  curent_valid_in : Inport  Port=5
  Add1 : Sum  Inputs=+-  RndMeth=Simplest  OutDataTypeStr=Inherit: Same as first input
  Add2 : Sum  Inputs=-+  RndMeth=Simplest  OutDataTypeStr=Inherit: Same as first input
  Add3 : Sum  RndMeth=Simplest  OutDataTypeStr=Inherit: Same as first input
  Compare To Constant : hdlsllib/Logic and Bit Operations/Compare To Constant  relop=>=  const=2*pi  OutDataTypeStr=boolean
      settings: SourceProductBaseCode=SL
  Compare To Constant1 : hdlsllib/Logic and Bit Operations/Compare To Constant  relop=<  const=0  OutDataTypeStr=boolean
      settings: SourceProductBaseCode=SL
  Constant : Constant  Value=2*pi  OutDataTypeStr=fixdt(1,18,14)  SampleTime=1.0000e-08
  Constant1 : Constant  Value=2*pi  OutDataTypeStr=fixdt(1,18,14)  SampleTime=1.0000e-08
  Data Type Conversion{1..14} (14 alike) : DataTypeConversion  OutDataTypeStr=fixdt(1,18,11)  SaturateOnIntegerOverflow=off  RndMeth=Floor
  Delay{,9..16} (9 alike) : Delay
  Delay{1..8,25} (9 alike) : Delay  DelayLength=1
  Delay{17..24,26} (9 alike) : Delay  DelayLength=3
  Demux : Demux  Outputs=3
  Demux1 : Demux  Outputs=3
  Detect Rise Positive : hdlsllib/Logic and Bit Operations/Detect Rise Positive  vinit=0  OutDataTypeStr=boolean
      settings: SourceProductBaseCode=SL
  Display : Display
  Display1 : Display
  Gain1 : Gain  Gain=1/(2*pi)  OutDataTypeStr=Inherit: Same as input  ParamDataTypeStr=Inherit: Same as input
  MATLAB Function : MATLAB Function  TreatAsAtomicUnit=on  SystemSampleTime=1/100000000
  Mux : Mux  Inputs=6
  Mux1 : Mux  Inputs=6
  Sine HDL Optimized1 : hdlsllib/Lookup Tables/Cosine HDL Optimized  OutputFormula=sin(2*pi*u) and cos(2*pi*u)  NumDataPoints=512  TableDataTypeStr=fixdt(1,15,14)  SimulateLUTROMDelay=off
      settings: SourceProductBaseCode=SL
  Switch : Switch  Criteria=u2 > Threshold  RndMeth=Simplest  SaturateOnIntegerOverflow=off  InputSameDT=off  OutDataTypeStr=Inherit: Same as first input
  Switch1 : Switch  Criteria=u2 > Threshold  RndMeth=Simplest  SaturateOnIntegerOverflow=off  InputSameDT=off  OutDataTypeStr=Inherit: Same as first input
  Switch_on{1..8} (8 alike) : Switch  Threshold=1  RndMeth=Simplest  SaturateOnIntegerOverflow=off  InputSameDT=off  OutDataTypeStr=Inherit: Same as first input
  datatyp_test : Scope  NumInputPorts=2
  i_ph_fixed_point : Scope  NumInputPorts=2
  i_alpha : Outport
  i_alpha_axi : Outport  Port=2
  i_beta : Outport  Port=3
  i_beta_axi : Outport  Port=4
  i_d : Outport  Port=5
  i_d_axi : Outport  Port=6
  i_q : Outport  Port=7
  i_q_axi : Outport  Port=8
  i_x : Outport  Port=9
  i_x_axi : Outport  Port=10
  i_y : Outport  Port=11
  i_y_axi : Outport  Port=12
  i_0_plus : Outport  Port=13
  i_0_plus_axi : Outport  Port=14
  i_0_minus : Outport  Port=15
  i_0_minus_axi : Outport  Port=16
  done : Outport  Port=17
  i_a1_axi : Outport  Port=18
  i_b1_axi : Outport  Port=19
  i_c1_axi : Outport  Port=20
  i_a2_axi : Outport  Port=21
  i_b2_axi : Outport  Port=22
  i_c2_axi : Outport  Port=23
  theta_test : Outport  Port=24
  wires:
  Delay8/1 -> Switch_on8/3
  Detect Rise Positive/1 -> Delay17/1, Switch_on7/2, Switch_on6/2, Switch_on1/2, Switch_on2/2, Switch_on3/2, Switch_on4/2, Switch_on5/2, Switch_on8/2  "End_Cycle"
  Delay4/1 -> Switch_on4/3
  Switch_on2/1 -> Delay2/1, i_c1_axi/1, Mux/3, Data Type Conversion3/1, MATLAB Function/3(i_c1)
  Delay1/1 -> Switch_on1/3
  Switch_on1/1 -> Delay1/1, i_b1_axi/1, Mux/2, Data Type Conversion2/1, MATLAB Function/2(i_b1)
  Switch_on6/1 -> i_a1_axi/1, Mux/1, Data Type Conversion9/1, MATLAB Function/1(i_a1), Delay6/1
  Switch_on4/1 -> Delay4/1, i_b2_axi/1, Mux/5, Data Type Conversion6/1, MATLAB Function/5(i_b2)
  curent_valid_in/1 -> Delay16/1  "End_Cycle"
  Switch/1 -> Switch1/3
  Switch_on3/1 -> i_a2_axi/1, Mux/4, Data Type Conversion4/1, MATLAB Function/4(i_a2), Delay3/1
  Delay6/1 -> Switch_on6/3
  Constant/1 -> Add2/1
  Add1/1 -> Switch/3, Compare To Constant1/1, Add3/1, Compare To Constant/1, Add2/2
  Delay2/1 -> Switch_on2/3
  Constant1/1 -> Add3/2
  theta_el/1 -> Delay14/1  "End_Cycle"
  Delay3/1 -> Switch_on3/3
  Add2/1 -> Switch/1
  Delay5/1 -> Switch_on5/3
  Add3/1 -> Switch1/1
  MATLAB Function/1(i_alpha) -> Data Type Conversion1/1  "curent_valid_in"
  MATLAB Function/2(i_beta) -> Data Type Conversion5/1  "curent_valid_in"
  MATLAB Function/3(i_x) -> Data Type Conversion8/1  "curent_valid_in"
  Compare To Constant/1 -> Switch/2
  Compare To Constant1/1 -> Switch1/2
  Delay25/1 -> Switch_on7/3
  theta_el_offset_/1 -> Delay15/1
  MATLAB Function/8(i_q) -> datatyp_test/1, Data Type Conversion14/1
  MATLAB Function/7(i_d) -> Data Type Conversion13/1
  MATLAB Function/6(i_0_minus) -> Data Type Conversion12/1
  MATLAB Function/5(i_0_plus) -> Data Type Conversion11/1
  MATLAB Function/4(i_y) -> Data Type Conversion10/1
  Switch_on5/1 -> Delay5/1, i_c2_axi/1, Data Type Conversion7/1, Mux/6, MATLAB Function/6(i_c2)
  Mux/1 -> i_ph_fixed_point/1
  Mux1/1 -> i_ph_fixed_point/2
  Data Type Conversion9/1 -> Mux1/1  "fc"
  Data Type Conversion2/1 -> Mux1/2  "fc"
  Data Type Conversion3/1 -> Mux1/3  "fc"
  Data Type Conversion4/1 -> Mux1/4  "fc"
  Data Type Conversion6/1 -> Mux1/5  "fc"
  Data Type Conversion7/1 -> Mux1/6  "fc"
  Data Type Conversion1/1 -> Delay18/1  "fc"
  Data Type Conversion5/1 -> Delay19/1  "fc"
  Data Type Conversion8/1 -> Delay20/1  "fc"
  Data Type Conversion10/1 -> Delay21/1  "fc"
  Data Type Conversion11/1 -> Delay22/1  "fc"
  Data Type Conversion12/1 -> Delay23/1  "fc"
  Data Type Conversion13/1 -> Delay24/1  "fc"
  Data Type Conversion14/1 -> datatyp_test/2, Delay26/1  "fc"
  Sine HDL Optimized1/1 -> Display1/1, MATLAB Function/7(sin_theta_el)
  Switch_on8/1 -> theta_test/1, Add1/1, Delay8/1
  Switch_on7/1 -> Add1/2, Delay25/1
  Gain1/1 -> Delay7/1
  Sine HDL Optimized1/2 -> MATLAB Function/8(cos_theta_el)
  Delay/1 -> Switch_on6/1
  Delay9/1 -> Switch_on1/1
  Delay10/1 -> Switch_on2/1
  Delay11/1 -> Switch_on3/1
  Delay12/1 -> Switch_on4/1
  Delay13/1 -> Switch_on5/1
  Delay14/1 -> Switch_on8/1
  Delay15/1 -> Switch_on7/1
  Delay16/1 -> Detect Rise Positive/1
  Delay17/1 -> done/1
  Delay18/1 -> i_alpha_axi/1, i_alpha/1
  Delay19/1 -> i_beta_axi/1, i_beta/1
  Delay20/1 -> i_x_axi/1, i_x/1
  Delay21/1 -> i_y_axi/1, i_y/1
  Delay22/1 -> i_0_plus_axi/1, i_0_plus/1
  Delay23/1 -> i_0_minus_axi/1, i_0_minus/1
  Delay24/1 -> i_d_axi/1, i_d/1
  Delay26/1 -> i_q_axi/1, i_q/1
  Switch1/1 -> Gain1/1  "End_Cycle"
  Delay7/1 -> Display/1, Sine HDL Optimized1/1
  abc_1/1 -> Demux/1  "End_Cycle"
  Demux/1 -> Delay/1
  Demux/2 -> Delay9/1
  Demux/3 -> Delay10/1
  abc_2/1 -> Demux1/1  "End_Cycle"
  Demux1/1 -> Delay11/1
  Demux1/2 -> Delay12/1
  Demux1/3 -> Delay13/1

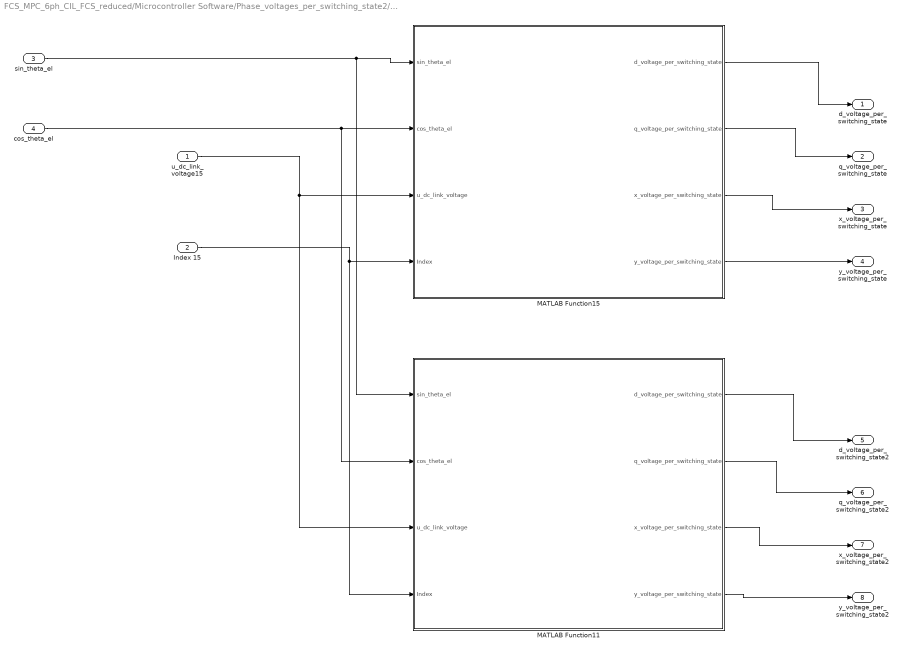
== system FCS_MPC_6ph_CIL_FCS_reduced/Microcontroller Software/Phase_voltages_per_switching_state2/Subsystem ==
  u_dc_link_voltage15 : Inport
  Index 15 : Inport  Port=2
  sin_theta_el : Inport  Port=3
  cos_theta_el : Inport  Port=4
  MATLAB Function11 : MATLAB Function  TreatAsAtomicUnit=on  SystemSampleTime=1/100000000
  MATLAB Function15 : MATLAB Function  TreatAsAtomicUnit=on  SystemSampleTime=1/100000000
  d_voltage_per_switching_state : Outport
  q_voltage_per_switching_state : Outport  Port=2
  x_voltage_per_switching_state : Outport  Port=3
  y_voltage_per_switching_state : Outport  Port=4
  d_voltage_per_switching_state2 : Outport  Port=5
  q_voltage_per_switching_state2 : Outport  Port=6
  x_voltage_per_switching_state2 : Outport  Port=7
  y_voltage_per_switching_state2 : Outport  Port=8
  wires:
  MATLAB Function11/4(y_voltage_per_switching_state) -> y_voltage_per_switching_state2/1
  MATLAB Function11/1(d_voltage_per_switching_state) -> d_voltage_per_switching_state2/1
  MATLAB Function15/2(q_voltage_per_switching_state) -> q_voltage_per_switching_state/1
  MATLAB Function11/3(x_voltage_per_switching_state) -> x_voltage_per_switching_state2/1
  MATLAB Function11/2(q_voltage_per_switching_state) -> q_voltage_per_switching_state2/1
  MATLAB Function15/1(d_voltage_per_switching_state) -> d_voltage_per_switching_state/1
  MATLAB Function15/4(y_voltage_per_switching_state) -> y_voltage_per_switching_state/1
  MATLAB Function15/3(x_voltage_per_switching_state) -> x_voltage_per_switching_state/1
  u_dc_link_voltage15/1 -> MATLAB Function11/3(u_dc_link_voltage), MATLAB Function15/3(u_dc_link_voltage)
  Index 15/1 -> MATLAB Function15/4(Index), MATLAB Function11/4(Index)
  sin_theta_el/1 -> MATLAB Function15/1(sin_theta_el), MATLAB Function11/1(sin_theta_el)
  cos_theta_el/1 -> MATLAB Function15/2(cos_theta_el), MATLAB Function11/2(cos_theta_el)

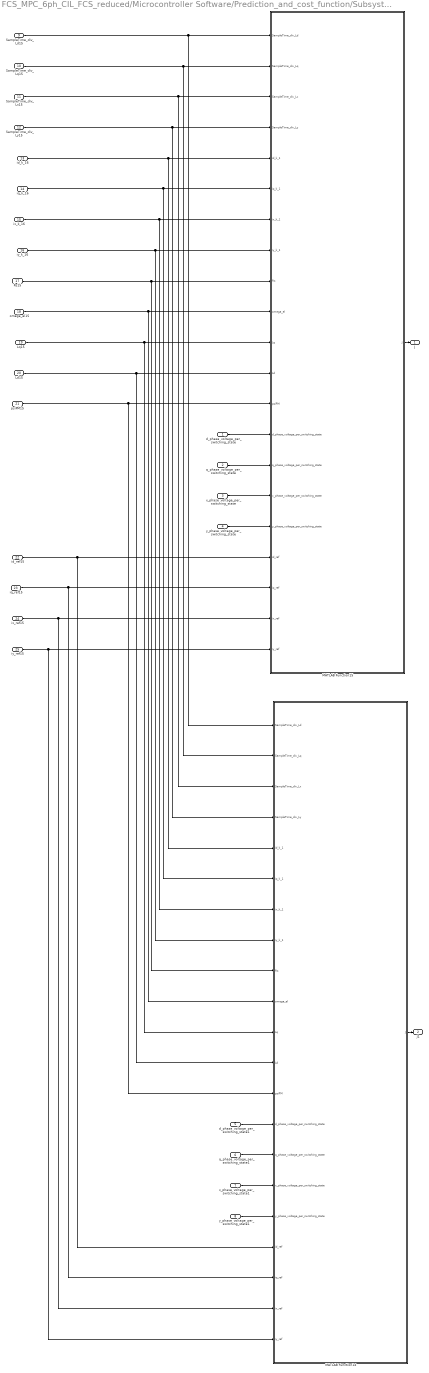
== system FCS_MPC_6ph_CIL_FCS_reduced/Microcontroller Software/Prediction_and_cost_function/Subsystem ==
  d_phase_voltage_per_switching_state : Inport
  q_phase_voltage_per_switching_state : Inport  Port=2
  x_phase_voltage_per_switching_state : Inport  Port=3
  y_phase_voltage_per_switching_state : Inport  Port=4
  d_phase_voltage_per_switching_state1 : Inport  Port=5
  q_phase_voltage_per_switching_state1 : Inport  Port=6
  x_phase_voltage_per_switching_state1 : Inport  Port=7
  y_phase_voltage_per_switching_state1 : Inport  Port=8
  SampleTime_div_Ld15 : Inport  Port=9
  SampleTime_div_Lq15 : Inport  Port=10
  SampleTime_div_Lx15 : Inport  Port=11
  SampleTime_div_Ly15 : Inport  Port=12
  id_k_16 : Inport  Port=13
  iq_k_16 : Inport  Port=14
  ix_k_16 : Inport  Port=15
  iy_k_16 : Inport  Port=16
  Rs15 : Inport  Port=17
  omega_el15 : Inport  Port=18
  Lq15 : Inport  Port=19
  Ld15 : Inport  Port=20
  psiPM15 : Inport  Port=21
  id_ref15 : Inport  Port=22
  iq_ref15 : Inport  Port=23
  ix_ref15 : Inport  Port=24
  iy_ref15 : Inport  Port=25
  MATLAB Function14 : MATLAB Function  TreatAsAtomicUnit=on  SystemSampleTime=1/100000000
  MATLAB Function15 : MATLAB Function  TreatAsAtomicUnit=on  SystemSampleTime=1/100000000
  J : Outport
  J1 : Outport  Port=2
  wires:
  q_phase_voltage_per_switching_state1/1 -> MATLAB Function14/15(q_phase_voltage_per_switching_state)
  SampleTime_div_Ld15/1 -> MATLAB Function14/1(SampleTime_div_Ld), MATLAB Function15/1(SampleTime_div_Ld)
  Rs15/1 -> MATLAB Function14/9(Rs), MATLAB Function15/9(Rs)
  y_phase_voltage_per_switching_state/1 -> MATLAB Function15/17(y_phase_voltage_per_switching_state)
  Lq15/1 -> MATLAB Function14/11(Lq), MATLAB Function15/11(Lq)
  d_phase_voltage_per_switching_state1/1 -> MATLAB Function14/14(d_phase_voltage_per_switching_state)
  x_phase_voltage_per_switching_state1/1 -> MATLAB Function14/16(x_phase_voltage_per_switching_state)
  iy_ref15/1 -> MATLAB Function14/21(iy_ref), MATLAB Function15/21(iy_ref)
  omega_el15/1 -> MATLAB Function14/10(omega_el), MATLAB Function15/10(omega_el)
  psiPM15/1 -> MATLAB Function14/13(psiPM), MATLAB Function15/13(psiPM)
  d_phase_voltage_per_switching_state/1 -> MATLAB Function15/14(d_phase_voltage_per_switching_state)
  y_phase_voltage_per_switching_state1/1 -> MATLAB Function14/17(y_phase_voltage_per_switching_state)
  MATLAB Function14/1(J) -> J1/1
  x_phase_voltage_per_switching_state/1 -> MATLAB Function15/16(x_phase_voltage_per_switching_state)
  SampleTime_div_Lx15/1 -> MATLAB Function14/3(SampleTime_div_Lx), MATLAB Function15/3(SampleTime_div_Lx)
  SampleTime_div_Ly15/1 -> MATLAB Function14/4(SampleTime_div_Ly), MATLAB Function15/4(SampleTime_div_Ly)
  SampleTime_div_Lq15/1 -> MATLAB Function14/2(SampleTime_div_Lq), MATLAB Function15/2(SampleTime_div_Lq)
  q_phase_voltage_per_switching_state/1 -> MATLAB Function15/15(q_phase_voltage_per_switching_state)
  MATLAB Function15/1(J) -> J/1
  ix_ref15/1 -> MATLAB Function14/20(ix_ref), MATLAB Function15/20(ix_ref)
  iq_ref15/1 -> MATLAB Function14/19(iq_ref), MATLAB Function15/19(iq_ref)
  id_ref15/1 -> MATLAB Function14/18(id_ref), MATLAB Function15/18(id_ref)
  Ld15/1 -> MATLAB Function14/12(Ld), MATLAB Function15/12(Ld)
  iy_k_16/1 -> MATLAB Function14/8(iy_k_1), MATLAB Function15/8(iy_k_1)
  ix_k_16/1 -> MATLAB Function14/7(ix_k_1), MATLAB Function15/7(ix_k_1)
  iq_k_16/1 -> MATLAB Function14/6(iq_k_1), MATLAB Function15/6(iq_k_1)
  id_k_16/1 -> MATLAB Function14/5(id_k_1), MATLAB Function15/5(id_k_1)

== matlab function FCS_MPC_6ph_CIL_FCS_reduced/Microcontroller Software/Switching_states/MATLAB Function1 ==
  data: I input; next_switching_state output
function next_switching_state = fcn(I)

    % Possible switching states of the 6-Phase 2-level inverter
    possible_swichting_states = [0	1	0	1	0	1	0	1	0	1	0	1;
                                
                                 1	0	1	0	1	0	0	1	0	1	0	1;
                                       
                                 1	0	0	1	0	1	1	0	0	1	0	1;
                                       
                                 1	0	1	0	0	1	1	0	0	1	0	1;
                                       
                                 0	1	1	0	0	1	0	1	1	0	0	1;
                                       
                                 0	1	1	0	1	0	0	1	1	0	0	1;
                                      
                                 0	1	1	0	0	1	1	0	1	0	0	1;
                                 1	0	1	0	0	1	1	0	1	0	0	1;
                                       
                                 0	1	0	1	1	0	0	1	0	1	1	0;
                                 1	0	0	1	1	0	0	1	0	1	1	0;
                                      
                                 1	0	0	1	0	1	1	0	0	1	1	0;
                                      
                                 1	0	0	1	1	0	1	0	0	1	1	0;
                                      
                                 0	1	0	1	1	0	0	1	1	0	1	0;
                                       
                                 0	1	1	0	1	0	0	1	1	0	1	0;
                                      
                                 0	1	0	1	0	1	1	0	1	0	1	0;
                                     
                                 1	0	1	0	1	0	1	0	1	0	1	0];

    % Initial condition
    if I==0
        I=int32(1);
    end

    % Output switching state
    next_switching_state=boolean(possible_swichting_states(I,:))';

end

== matlab function FCS_MPC_6ph_CIL_FCS_reduced/6ph_PMSM_30deg_VSD1 ==
  data: u1 input; y1 output; u2 input; u3 input; u4 input; u5 input; u6 input; y2 output; y3 output; y4 output; y5 output; y6 output; k6 input; c6 input
function [y1,y2,y3,y4,y5,y6] = VSD_asymm_30(u1,u2,u3,u4,u5,u6,k6,c6)

A =single([0 0 0 0 0 0]');

A =    k6*[1    -0.5        -0.5        sqrt(3)/2   -sqrt(3)/2  0 ;
           0    sqrt(3)/2   -sqrt(3)/2  0.5         0.5         -1;
           1    -0.5        -0.5        -sqrt(3)/2  sqrt(3)/2   0 ;
           0    -sqrt(3)/2  sqrt(3)/2   0.5         0.5         -1;
           c6   c6          c6          0           0           0 ;
           0    0           0           c6          c6          c6] * [u1 u2 u3 u4 u5 u6]';

y1 =single(A(1));
y2 =single(A(2));
y3 =single(A(3));
y4 =single(A(4));
y5 =single(A(5));
y6 =single(A(6));

== matlab function FCS_MPC_6ph_CIL_FCS_reduced/Microcontroller Software/Prediction_and_cost_function/Subsystem/MATLAB Function14 ==
  data: SampleTime_div_Ld input; J output; SampleTime_div_Lq input; SampleTime_div_Lx input; SampleTime_div_Ly input; id_k_1 input; iq_k_1 input; ix_k_1 input; iy_k_1 input; Rs input; omega_el input; Lq input; Ld input; psiPM input; d_phase_voltage_per_switching_state input; q_phase_voltage_per_switching_state input; x_phase_voltage_per_switching_state input; y_phase_voltage_per_switching_state input; id_ref input; iq_ref input; ix_ref input; iy_ref input
function J = fcn(SampleTime_div_Ld, SampleTime_div_Lq, SampleTime_div_Lx, SampleTime_div_Ly, id_k_1, iq_k_1, ix_k_1, iy_k_1, Rs, omega_el, Lq, Ld, psiPM, d_phase_voltage_per_switching_state, q_phase_voltage_per_switching_state, x_phase_voltage_per_switching_state, y_phase_voltage_per_switching_state, id_ref, iq_ref, ix_ref, iy_ref)
     
        % Prediction of the d-, q-, x-, y-currents of the 6-Phase-PMSM with the finite control set 
        id_k_2 = single(SampleTime_div_Ld*(d_phase_voltage_per_switching_state-id_k_1*Rs+omega_el*Lq*iq_k_1)+id_k_1);
        iq_k_2 = single(SampleTime_div_Lq*(q_phase_voltage_per_switching_state-iq_k_1*Rs-omega_el*(psiPM+id_k_1*Ld))+iq_k_1);
        ix_k_2 = single(SampleTime_div_Lx*(x_phase_voltage_per_switching_state-ix_k_1*Rs)+ix_k_1);
        iy_k_2 = single(SampleTime_div_Ly*(y_phase_voltage_per_switching_state-iy_k_1*Rs)+iy_k_1);
        
        % Calculation of the cost function
        J = single((id_ref-id_k_2)^2+(iq_ref-iq_k_2)^2+(ix_ref-ix_k_2)^2+(iy_ref-iy_k_2)^2);
      

end
